simulink model "Robot_Phase1_PASS"  (R2026a)
settings: Solver=ode15s  StopTime=20  FixedStep=0.001  MaxStep=0.01  AbsTol=1e-6
model workspace: external: MATLAB File GDOFrobot_DataFile.m (data not in the file)
values from neighbouring files (symbols this model uses):
  enc_noise_signal = randn(length(t_noise), 3)    [generate_dataset_v2.m]
  N = size(residual, 1)    [extract_features.m]    (also in extract_features_windowed.m)
  t_noise = (0:dt_noise:sim_duration)'    [generate_dataset_v2.m]
  Y = categorical(label_vector)    [SVM_classifier_training.m]
undefined symbols (not defined in the file or in its folder): BEAR_PARAMS, DEG_INDEX, ENC_PARAMS, FAULT_JOINT, FAULT_TYPE, GEAR_PARAMS, IMB_PARAMS, sim_payload_mass, smiData, X, Z
libraries: sm_lib x42, nesl_utility x20, simulink x3
(part 1 of 2)
settings Model: Creator=AMMAR  LastModifiedBy=mkame
settings DebuggingCC: InheritedTsInSrcMsg=none
settings ExplorerConfigSet: InternalSimMechanicsExplorerSettings=|
  | <ExplorerConfiguration>
  | 
  |   <canonicalview>default</canonicalview>
  | 
  |   <TilePanel>
  |     <TileInfo>
  |       <Tiles Columns="1" Count="1" Height="465" Rows="1" Width="822">
  |         <Row Weight="1"/>
  |         <Column Weight="1"/>
  |         <Tile Height="1" Width="1" X="0" Y="0"/>
  |       </Tiles>
  |     </TileInfo>
  |     <SceneInfo>
  |       <SceneViewer>
  |         <IsThisViewStd>
  |           <IsStandardView>off</IsStandardView>
  |           <StandardViewName>Front</StandardViewName>
  |         </IsThisViewStd>
  |         <BGColor>
  |           <R>1</R>
  |           <G>1</G>
  |           <B>1</B>
  |           <A>1</A>
  |         </BGColor>
  |         <Camera>
  |           <DoPerspective>off</DoPerspective>
  |           <Position>
  |             <X>-2.8828618955433565</X>
  |             <Y>-1.823236819125285</Y>
  |             <Z>0.92007110645659929</Z>
  |           </Position>
  |           <Center>
  |             <X>-0.4974271117814994</X>
  |             <Y>-0.23235959407589699</Y>
  |             <Z>0.46408144410745272</Z>
  |           </Center>
  |           <Up>
  |             <X>0.126273929236871</X>
  |             <Y>0.093720705637387533</Y>
  |             <Z>0.98755826366342159</Z>
  |           </Up>
  |           <XLim>0.50845975031305723</XLim>
  |           <YLim>0.50845975031305723</YLim>
  |           <ViewLimDist>0.01</ViewLimDist>
  |         </Camera>
  |       </SceneViewer>
  |     </SceneInfo>
  |   </TilePanel>
  | 
  |   <MechEditorPanel>
  |     <GfxPanelCameraMap/>
  |     <Cameras/>
  |     <VideoCreator>
  |       <IncludeTiles>All</IncludeTiles>
  |       <IncludeTime>on</IncludeTime>
  |       <IncludeWorldFrame>off</IncludeWorldFrame>
  |       <PlaybackSpeedRatio>1</PlaybackSpeedRatio>
  |       <FrameRate>30</FrameRate>
  |       <FrameSize>auto</FrameSize>
  |       <VideoFormat>UncompressedAVI</VideoFormat>
  |     </VideoCreator>
  |   </MechEditorPanel>
  | 
  |   <PlaybackSettings>
  |     <PlaybackSpeedFactor>2</PlaybackSpeedFactor>
  |   </PlaybackSettings>
  | 
  | </ExplorerConfiguration>

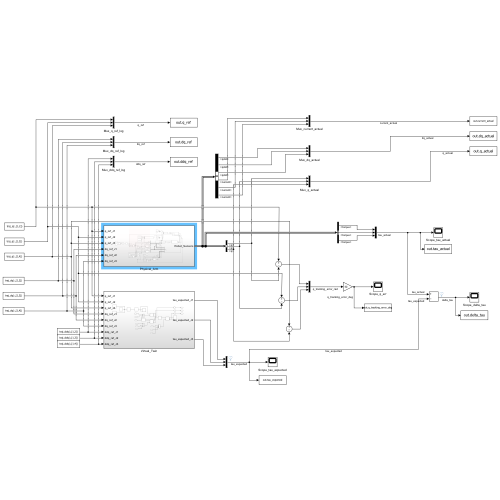
[thumbnail: Simulink's stored preview of the top-level diagram]
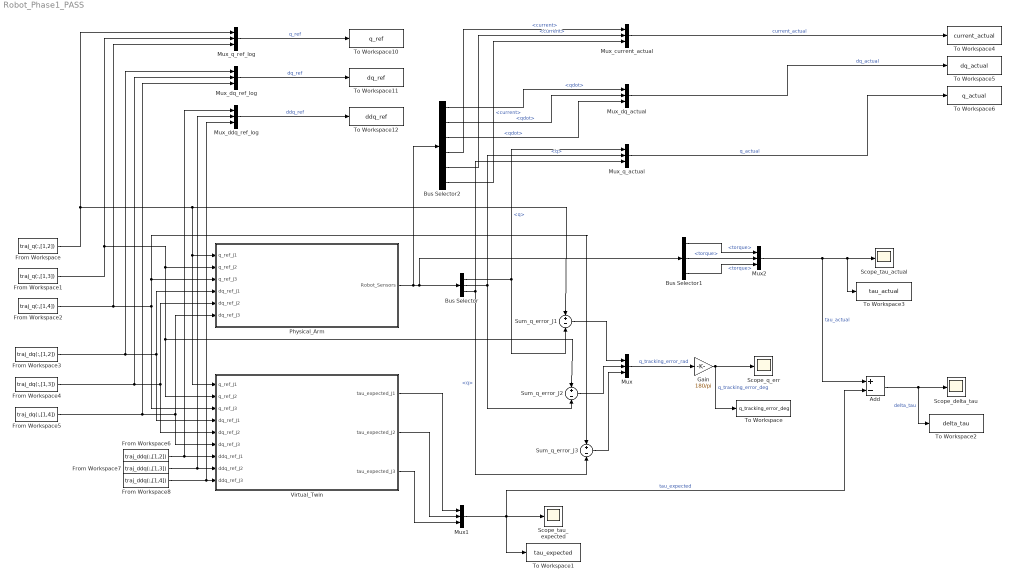
== system Robot_Phase1_PASS ==
  Add : Sum  Inputs=+-
  Bus Selector : BusSelector  OutputSignals=Joint1_Signals.q,Joint2_Signals.q,Joint3_Signals.q
  Bus Selector1 : BusSelector  OutputSignals=Joint1_Signals.torque,Joint2_Signals.torque,Joint3_Signals.torque
  Bus Selector2 : BusSelector  OutputSignals=Joint1_Signals.qdot,Joint2_Signals.qdot,Joint3_Signals.qdot,Joint1_Signals.current,Joint2_Signals.current,Joint3_Signals.current
  From Workspace : FromWorkspace  VariableName=traj_q(:,[1,2])  SampleTime=-1
  From Workspace1 : FromWorkspace  VariableName=traj_q(:,[1,3])  SampleTime=-1
  From Workspace2 : FromWorkspace  VariableName=traj_q(:,[1,4])  SampleTime=-1
  From Workspace3 : FromWorkspace  VariableName=traj_dq(:,[1,2])  SampleTime=-1
  From Workspace4 : FromWorkspace  VariableName=traj_dq(:,[1,3])  SampleTime=-1
  From Workspace5 : FromWorkspace  VariableName=traj_dq(:,[1,4])  SampleTime=-1
  From Workspace6 : FromWorkspace  VariableName=traj_ddq(:,[1,2])  SampleTime=-1
  From Workspace7 : FromWorkspace  VariableName=traj_ddq(:,[1,3])  SampleTime=-1
  From Workspace8 : FromWorkspace  VariableName=traj_ddq(:,[1,4])  SampleTime=-1
  Gain : Gain  Gain=180/pi
  Mux : Mux  Inputs=3
  Mux1 : Mux  Inputs=3
  Mux2 : Mux  Inputs=3
  Mux_current_actual : Mux  Inputs=3
  Mux_ddq_ref_log : Mux  Inputs=3
  Mux_dq_actual : Mux  Inputs=3
  Mux_dq_ref_log : Mux  Inputs=3
  Mux_q_actual : Mux  Inputs=3
  Mux_q_ref_log : Mux  Inputs=3
  Physical_Arm : Subsystem
  Scope_delta_tau : Scope
      settings: ActiveDisplayYMinimum=-2.4660979772206608  ActiveDisplayYMaximum=7.674798064954345  DataLoggingVariableName=ScopeData2
  Scope_q_err : Scope
      settings: ActiveDisplayYMinimum=-97.469420637848955  ActiveDisplayYMaximum=96.880109513754348
  Scope_tau_actual : Scope
      settings: ActiveDisplayYMinimum=-1  ActiveDisplayYMaximum=1  DataLoggingVariableName=ScopeData3
  Scope_tau_expected : Scope
      settings: ActiveDisplayYMinimum=-15.168732068313531  ActiveDisplayYMaximum=6.028938661872969
  "Sum_q_error_J1 " : Sum  Inputs=+-
  Sum_q_error_J2 : Sum  Inputs=+-
  Sum_q_error_J3 : Sum  Inputs=+-
  To Workspace : ToWorkspace  VariableName=q_tracking_error_deg  SaveFormat=Timeseries  SampleTime=-1
  To Workspace1 : ToWorkspace  VariableName=tau_expected  SaveFormat=Timeseries  SampleTime=-1
  To Workspace10 : ToWorkspace  VariableName=q_ref  SaveFormat=Timeseries  SampleTime=-1
  To Workspace11 : ToWorkspace  VariableName=dq_ref  SaveFormat=Timeseries  SampleTime=-1
  To Workspace12 : ToWorkspace  VariableName=ddq_ref  SaveFormat=Timeseries  SampleTime=-1
  To Workspace2 : ToWorkspace  VariableName=delta_tau  SaveFormat=Timeseries  SampleTime=-1
  To Workspace3 : ToWorkspace  VariableName=tau_actual  SaveFormat=Timeseries  SampleTime=-1
  To Workspace4 : ToWorkspace  VariableName=current_actual  SaveFormat=Timeseries  SampleTime=-1
  To Workspace5 : ToWorkspace  VariableName=dq_actual  SaveFormat=Timeseries  SampleTime=-1
  To Workspace6 : ToWorkspace  VariableName=q_actual  SaveFormat=Timeseries  SampleTime=-1
  Virtual_Twin : Subsystem
  wires:
  From Workspace/1 -> Mux_q_ref_log/1, Virtual_Twin/1("q_ref_J1 "), Physical_Arm/1("q_ref_J1  "), "Sum_q_error_J1 "/1
  From Workspace4/1 -> Mux_dq_ref_log/2, Physical_Arm/5(dq_ref_J2), Virtual_Twin/5(dq_ref_J2)
  From Workspace7/1 -> Mux_ddq_ref_log/2, Virtual_Twin/8(ddq_ref_J2)
  From Workspace1/1 -> Mux_q_ref_log/2, Virtual_Twin/2(q_ref_J2), Sum_q_error_J2/1, Physical_Arm/2(q_ref_J2)
  From Workspace5/1 -> Mux_dq_ref_log/3, Physical_Arm/6(dq_ref_J3), Virtual_Twin/6(dq_ref_J3)
  From Workspace3/1 -> Mux_dq_ref_log/1, Physical_Arm/4(dq_ref_J1), Virtual_Twin/4(dq_ref_J1)
  From Workspace2/1 -> Mux_q_ref_log/3, Sum_q_error_J3/1, Physical_Arm/3(q_ref_J3), Virtual_Twin/3(q_ref_J3)
  From Workspace6/1 -> Mux_ddq_ref_log/1, Virtual_Twin/7(ddq_ref_J1)
  From Workspace8/1 -> Mux_ddq_ref_log/3, Virtual_Twin/9(ddq_ref_J3)
  Physical_Arm/1(Robot_Sensors) -> Bus Selector2/1, Bus Selector1/1, Bus Selector/1
  Bus Selector/1 -> Mux_q_actual/1, "Sum_q_error_J1 "/2  "<q>"
  "Sum_q_error_J1 "/1 -> Mux/1
  Sum_q_error_J2/1 -> Mux/2
  Sum_q_error_J3/1 -> Mux/3
  Mux/1 -> Gain/1  "q_tracking_error_rad"
  Gain/1 -> To Workspace/1, Scope_q_err/1  "q_tracking_error_deg"
  Bus Selector/2 -> Mux_q_actual/2, Sum_q_error_J2/2  "<q>"
  Bus Selector/3 -> Mux_q_actual/3, Sum_q_error_J3/2  "<q>"
  Virtual_Twin/1(tau_expected_J1) -> Mux1/1
  Virtual_Twin/2(tau_expected_J2) -> Mux1/2
  Virtual_Twin/3(tau_expected_J3) -> Mux1/3
  Mux1/1 -> To Workspace1/1, Add/2, Scope_tau_expected/1  "tau_expected"
  Bus Selector1/1 -> Mux2/1  "<torque>"
  Bus Selector1/2 -> Mux2/2  "<torque>"
  Bus Selector1/3 -> Mux2/3  "<torque>"
  Mux2/1 -> Add/1, To Workspace3/1, Scope_tau_actual/1  "tau_actual"
  Add/1 -> To Workspace2/1, Scope_delta_tau/1  "delta_tau"
  Bus Selector2/1 -> Mux_dq_actual/1  "<qdot>"
  Bus Selector2/2 -> Mux_dq_actual/2  "<qdot>"
  Bus Selector2/3 -> Mux_dq_actual/3  "<qdot>"
  Bus Selector2/4 -> Mux_current_actual/1  "<current>"
  Bus Selector2/5 -> Mux_current_actual/2  "<current>"
  Bus Selector2/6 -> Mux_current_actual/3  "<current>"
  Mux_current_actual/1 -> To Workspace4/1  "current_actual"
  Mux_dq_actual/1 -> To Workspace5/1  "dq_actual"
  Mux_q_actual/1 -> To Workspace6/1  "q_actual"
  Mux_q_ref_log/1 -> To Workspace10/1  "q_ref"
  Mux_dq_ref_log/1 -> To Workspace11/1  "dq_ref"
  Mux_ddq_ref_log/1 -> To Workspace12/1  "ddq_ref"

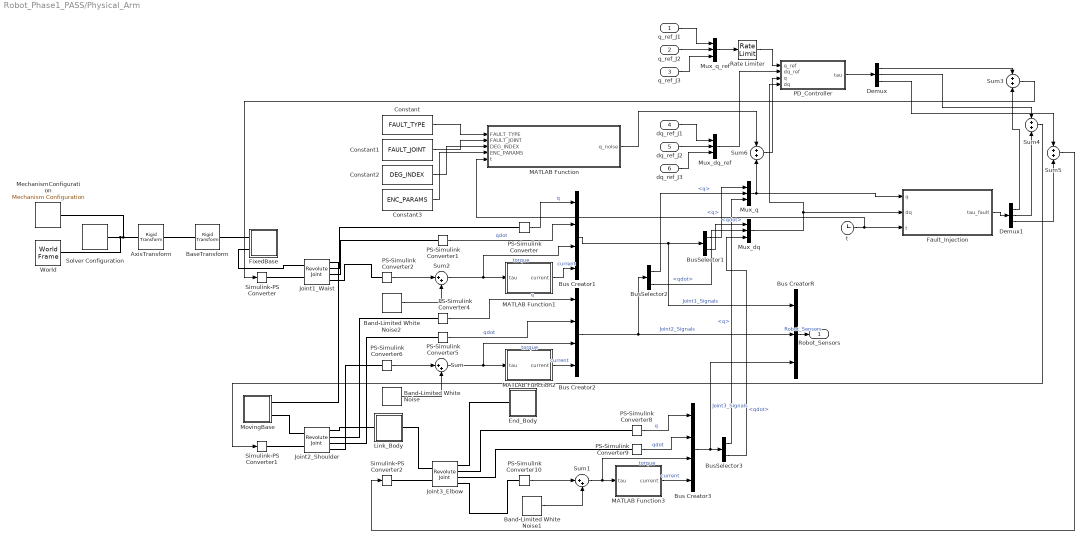
== system Robot_Phase1_PASS/Physical_Arm ==
  "q_ref_J1  " : Inport
  q_ref_J2 : Inport  Port=2
  q_ref_J3 : Inport  Port=3
  dq_ref_J1 : Inport  Port=4
  dq_ref_J2 : Inport  Port=5
  dq_ref_J3 : Inport  Port=6
  AxisTransform : sm_lib/Frames and Transforms/Rigid Transform  RotationMethod=StandardAxis  FollAlignAxisA=+X  BaseAlignAxisA=+Y  FollAlignAxisB=+Y  BaseAlignAxisB=+Z  RotationStandardAxis=+X  RotationAngle=pi/2  RotationAngleUnits=rad  RotationArbitraryAxis=[0 0 1]  RotationSequenceAxes=FollowerAxes  RotationSequence=XYX  RotationSequenceAngles=[0 0 0]  RotationSequenceAnglesUnits=deg  RotationMatrix=[1 0 0;0 1 0;0 0 1]  Quaternion=[1 0 0 0]  TranslationMethod=None  TranslationCartesianOffset=[0 0 0]  TranslationCartesianOffsetUnits=m  TranslationStandardAxis=+Z  TranslationStandardOffset=0  TranslationStandardOffsetUnits=m  TranslationROffset=0  TranslationROffsetUnits=m  TranslationThetaOffset=0  TranslationThetaOffsetUnits=deg  TranslationZOffset=0  TranslationZOffsetUnits=m
  Band-Limited White Noise : simulink/Sources/Band-Limited White Noise  Cov=[1e-7]  Ts=0.001  seed=[23342]
  Band-Limited White Noise1 : simulink/Sources/Band-Limited White Noise  Cov=[1e-7]  Ts=0.001  seed=[23343]
  Band-Limited White Noise2 : simulink/Sources/Band-Limited White Noise  Cov=[1e-7]  Ts=0.001  seed=[23341]
  BaseTransform : sm_lib/Frames and Transforms/Rigid Transform  RotationMethod=ArbitraryAxis  FollAlignAxisA=+X  BaseAlignAxisA=+Y  FollAlignAxisB=+Y  BaseAlignAxisB=+Z  RotationStandardAxis=+X  RotationAngle=smiData.RigidTransform(7).angle  RotationAngleUnits=rad  RotationArbitraryAxis=smiData.RigidTransform(7).axis  RotationSequenceAxes=FollowerAxes  RotationSequence=XYX  RotationSequenceAngles=[0 0 0]  RotationSequenceAnglesUnits=deg  RotationMatrix=[1 0 0;0 1 0;0 0 1]  Quaternion=[1 0 0 0]  TranslationMethod=Cartesian  TranslationCartesianOffset=smiData.RigidTransform(7).translation  TranslationCartesianOffsetUnits=mm  TranslationStandardAxis=+Z  TranslationStandardOffset=0.75  TranslationStandardOffsetUnits=m  TranslationROffset=0  TranslationROffsetUnits=m  TranslationThetaOffset=0  TranslationThetaOffsetUnits=deg  TranslationZOffset=0  TranslationZOffsetUnits=m
  Bus Creator1 : BusCreator  Inputs=4
  Bus Creator2 : BusCreator  Inputs=4
  Bus Creator3 : BusCreator  Inputs=4
  Bus CreatorR : BusCreator  Inputs=3
  BusSelector1 : BusSelector  OutputSignals=q,qdot
  BusSelector2 : BusSelector  OutputSignals=q,qdot
  BusSelector3 : BusSelector  OutputSignals=q,qdot
  Constant : Constant  Value=FAULT_TYPE
  Constant1 : Constant  Value=FAULT_JOINT
  Constant2 : Constant  Value=DEG_INDEX
  Constant3 : Constant  Value=ENC_PARAMS
  Demux : Demux  Outputs=3
  Demux1 : Demux  Outputs=3
  End_Body : Subsystem
  Fault_Injection : Subsystem
  FixedBase : Subsystem
  Joint1_Waist : sm_lib/Joints/Revolute Joint  JointMode=Normal  CompositeWrenchDir=FollowerOnBase  CompositeWrenchFrame=BaseFrame  SenseConstraintForce=off  SenseConstraintTorque=off  SenseTotalForce=off  SenseTotalTorque=off  PositionTargetSpecify=on  PositionTargetPriority=High  PositionTargetValue=0  PositionTargetValueUnits=rad  VelocityTargetSpecify=on  VelocityTargetPriority=High  VelocityTargetValue=0  VelocityTargetValueUnits=deg/s  EquilibriumPosition=0  EquilibriumPositionUnits=deg  SpringStiffness=0  SpringStiffnessUnits=N*m/deg  DampingCoefficient=1  DampingCoefficientUnits=N*m*s/rad  LowerLimitSpecify=on  LowerLimitBound=-180  LowerLimitBoundUnits=deg  LowerLimitStiffness=1e4  LowerLimitStiffnessUnits=N*m/deg  LowerLimitDamping=10  LowerLimitDampingUnits=N*m/(deg/s)  LowerLimitTransitionRegionWidth=0.1  LowerLimitTransitionRegionWidthUnits=deg  UpperLimitSpecify=on  UpperLimitBound=180  UpperLimitBoundUnits=deg  UpperLimitStiffness=1e4  UpperLimitStiffnessUnits=N*m/deg  UpperLimitDamping=10  UpperLimitDampingUnits=N*m/(deg/s)  UpperLimitTransitionRegionWidth=0.1  UpperLimitTransitionRegionWidthUnits=deg  TorqueActuationMode=InputTorque  MotionActuationMode=ComputedMotion  SensePosition=on  SenseVelocity=on  SenseAcceleration=off  SenseTorqueForce=on  SenseLowerLimitTorqueForce=off  SenseUpperLimitTorqueForce=off
  Joint2_Shoulder : sm_lib/Joints/Revolute Joint  JointMode=Normal  CompositeWrenchDir=FollowerOnBase  CompositeWrenchFrame=BaseFrame  SenseConstraintForce=off  SenseConstraintTorque=off  SenseTotalForce=off  SenseTotalTorque=off  PositionTargetSpecify=on  PositionTargetPriority=High  PositionTargetValue=-pi/4  PositionTargetValueUnits=rad  VelocityTargetSpecify=on  VelocityTargetPriority=High  VelocityTargetValue=0  VelocityTargetValueUnits=deg/s  EquilibriumPosition=0  EquilibriumPositionUnits=deg  SpringStiffness=0  SpringStiffnessUnits=N*m/deg  DampingCoefficient=1.5  DampingCoefficientUnits=N*m*s/rad  LowerLimitSpecify=on  LowerLimitBound=-195  LowerLimitBoundUnits=deg  LowerLimitStiffness=1e4  LowerLimitStiffnessUnits=N*m/deg  LowerLimitDamping=10  LowerLimitDampingUnits=N*m/(deg/s)  LowerLimitTransitionRegionWidth=0.1  LowerLimitTransitionRegionWidthUnits=deg  UpperLimitSpecify=on  UpperLimitBound=-15  UpperLimitBoundUnits=deg  UpperLimitStiffness=1e4  UpperLimitStiffnessUnits=N*m/deg  UpperLimitDamping=10  UpperLimitDampingUnits=N*m/(deg/s)  UpperLimitTransitionRegionWidth=0.1  UpperLimitTransitionRegionWidthUnits=deg  TorqueActuationMode=InputTorque  MotionActuationMode=ComputedMotion  SensePosition=on  SenseVelocity=on  SenseAcceleration=off  SenseTorqueForce=on  SenseLowerLimitTorqueForce=off  SenseUpperLimitTorqueForce=off
  Joint3_Elbow : sm_lib/Joints/Revolute Joint  JointMode=Normal  CompositeWrenchDir=FollowerOnBase  CompositeWrenchFrame=BaseFrame  SenseConstraintForce=off  SenseConstraintTorque=off  SenseTotalForce=off  SenseTotalTorque=off  PositionTargetSpecify=on  PositionTargetPriority=High  PositionTargetValue=-pi/4  PositionTargetValueUnits=rad  VelocityTargetSpecify=on  VelocityTargetPriority=High  VelocityTargetValue=0  VelocityTargetValueUnits=deg/s  EquilibriumPosition=0  EquilibriumPositionUnits=deg  SpringStiffness=0  SpringStiffnessUnits=N*m/deg  DampingCoefficient=0.5  DampingCoefficientUnits=N*m*s/rad  LowerLimitSpecify=on  LowerLimitBound=-165  LowerLimitBoundUnits=deg  LowerLimitStiffness=1e4  LowerLimitStiffnessUnits=N*m/deg  LowerLimitDamping=10  LowerLimitDampingUnits=N*m/(deg/s)  LowerLimitTransitionRegionWidth=0.1  LowerLimitTransitionRegionWidthUnits=deg  UpperLimitSpecify=on  UpperLimitBound=60  UpperLimitBoundUnits=deg  UpperLimitStiffness=1e4  UpperLimitStiffnessUnits=N*m/deg  UpperLimitDamping=10  UpperLimitDampingUnits=N*m/(deg/s)  UpperLimitTransitionRegionWidth=0.1  UpperLimitTransitionRegionWidthUnits=deg  TorqueActuationMode=InputTorque  MotionActuationMode=ComputedMotion  SensePosition=on  SenseVelocity=on  SenseAcceleration=off  SenseTorqueForce=on  SenseLowerLimitTorqueForce=off  SenseUpperLimitTorqueForce=off
  Link_Body : Subsystem
  MATLAB Function : MATLAB Function  TreatAsAtomicUnit=on
  MATLAB Function1 : MATLAB Function  TreatAsAtomicUnit=on
  MATLAB Function2 : MATLAB Function  TreatAsAtomicUnit=on
  MATLAB Function3 : MATLAB Function  TreatAsAtomicUnit=on
  MechanismConfiguration : sm_lib/Utilities/Mechanism Configuration  UniformGravity=Constant  GravityVector=[0 0 -9.80665]  GravityVectorUnits=m/s^2  LinearizationDelta=0.001  JointModeTransitionNonlinearIterations=2
  MovingBase : Subsystem
  "Mux_dq   " : Mux  Inputs=3
  "Mux_dq_ref " : Mux  Inputs=3
  "Mux_q    " : Mux  Inputs=3
  "Mux_q_ref  " : Mux  Inputs=3
  PD_Controller : Subsystem
  PS-Simulink Converter : nesl_utility/PS-Simulink Converter  PhysicalDomain=network_engine_domain  SubClassName=ps_output  LeftPortType=input  RightPortType=output  PseudoPeriodic=off  Frequencies=[]  VectorFormat=inherit  Unit=rad  AffineConversion=off
  PS-Simulink Converter{1..2,5..6,9..10} (6 alike) : nesl_utility/PS-Simulink Converter  PhysicalDomain=network_engine_domain  SubClassName=ps_output  LeftPortType=input  RightPortType=output  PseudoPeriodic=off  Frequencies=[]  VectorFormat=inherit  Unit=inherit  AffineConversion=off
  PS-Simulink Converter4 : nesl_utility/PS-Simulink Converter  PhysicalDomain=network_engine_domain  SubClassName=ps_output  LeftPortType=input  RightPortType=output  PseudoPeriodic=off  Frequencies=[]  VectorFormat=inherit  Unit=rad  AffineConversion=off
  PS-Simulink Converter8 : nesl_utility/PS-Simulink Converter  PhysicalDomain=network_engine_domain  SubClassName=ps_output  LeftPortType=input  RightPortType=output  PseudoPeriodic=off  Frequencies=[]  VectorFormat=inherit  Unit=rad  AffineConversion=off
  Rate Limiter : RateLimiter  RisingSlewLimit=10  FallingSlewLimit=-10  SampleTimeMode=inherited
  Simulink-PS Converter : nesl_utility/Simulink-PS Converter  PhysicalDomain=network_engine_domain  SubClassName=ps_input  LeftPortType=input  RightPortType=output  PseudoPeriodic=off  Frequencies=[]  NoiseDistribution=none  NoiseParameters=[]  Unit=N*m  AffineConversion=off  FilteringAndDerivatives=provide  SimscapeFilterOrder=1  InputFilterTimeConstant=0.001  UdotUserProvided=0
  Simulink-PS Converter1 : nesl_utility/Simulink-PS Converter  PhysicalDomain=network_engine_domain  SubClassName=ps_input  LeftPortType=input  RightPortType=output  PseudoPeriodic=off  Frequencies=[]  NoiseDistribution=none  NoiseParameters=[]  Unit=N*m  AffineConversion=off  FilteringAndDerivatives=provide  SimscapeFilterOrder=1  InputFilterTimeConstant=0.001  UdotUserProvided=0
  Simulink-PS Converter2 : nesl_utility/Simulink-PS Converter  PhysicalDomain=network_engine_domain  SubClassName=ps_input  LeftPortType=input  RightPortType=output  PseudoPeriodic=off  Frequencies=[]  NoiseDistribution=none  NoiseParameters=[]  Unit=N*m  AffineConversion=off  FilteringAndDerivatives=provide  SimscapeFilterOrder=1  InputFilterTimeConstant=0.001  UdotUserProvided=0
  Solver Configuration : nesl_utility/Solver Configuration  PhysicalDomain=network_engine_domain  SubClassName=solver  LeftPortType=input  RightPortType=generic  Tones=[]  Harmonics=[]  SimulateNoise=off  Profile=off  UseLocalSampling=off  EnableSwitchedLinearOptims=on  FrequencyDomain=off  UseCCode=off  RelTol=0.001  AbsTol=0.001  MinStep=1e-09  ToWorkspace=off  RevertToSquareIcSolve=off  NumHomotopyIterations=100  PhasorMode=off  PhasorModeNumHarmonics=1  ConsistencySolver=NEWTON_XTOL_AFTER_FTOL  CanonicalOrdering=CANONICAL  OptimizeIntermediates=OPTIMIZED  IndexReductionMethod=DerivativeReplacement  DoDC=off  ResidualTolerance=1e-09  ConsistencyTolSource=GLOBAL  ConsistencyAbsTol=0.001  ConsistencyRelTol=0.001  ConsistencyTolFactor=0.001  UseLocalSolver=off  LocalSolverChoice=NE_BACKWARD_EULER_ADVANCER  ResolveIndetEquations=on  FunctionEvalNumThread=1  LocalSolverSampleTime=0.001  DoFixedCost=off  MaxNonlinIter=3  MaxModeIter=2  ComputeImpulses=off  ImpulseIterations=2  LinearAlgebra=auto  LinearAlgebraNumThread=0  EquationFormulation=NE_TIME_EF  DelaysMemoryBudget=1024  AutomaticFiltering=on  FilteringTimeConstant=0.001  PartitionStorageMethod=AS_NEEDED  PartitionMemoryBudget=1024  PartitionMethod=ROBUST  MultibodyUseLocalSolver=off  MultibodyLocalSolverChoice=ODE1  MultibodyLocalSolverSampleTime=0.001
  Sum : Sum  Inputs=|++
  Sum1 : Sum  Inputs=|++
  Sum2 : Sum  Inputs=|++
  Sum{3..6} (4 alike) : Sum
  World : sm_lib/Frames and Transforms/World Frame
  t : Clock
  Robot_Sensors : Outport
  wires:
  PD_Controller/1(tau) -> Demux/1
  Sum1/1 -> Bus Creator3/3, MATLAB Function3/1(tau)  "torque"
  MATLAB Function2/1(current) -> Bus Creator2/4  "current"
  BusSelector2/2 -> "Mux_dq   "/2  "<qdot>"
  PS-Simulink Converter9/1 -> Bus Creator3/2  "qdot"
  PS-Simulink Converter6/1 -> Sum/1
  Bus Creator2/1 -> BusSelector2/1, Bus CreatorR/2  "Joint2_Signals"
  Rate Limiter/1 -> PD_Controller/1(q_ref)
  Sum2/1 -> Bus Creator1/3, MATLAB Function1/1(tau)  "torque"
  Bus Creator1/1 -> BusSelector1/1, Bus CreatorR/1  "Joint1_Signals"
  BusSelector3/1 -> "Mux_q    "/3  "<q>"
  PS-Simulink Converter2/1 -> Sum2/1
  MATLAB Function1/1(current) -> Bus Creator1/4  "current"
  BusSelector1/2 -> "Mux_dq   "/1  "<qdot>"
  BusSelector1/1 -> "Mux_q    "/1  "<q>"
  Sum/1 -> Bus Creator2/3, MATLAB Function2/1(tau)  "torque"
  PS-Simulink Converter1/1 -> Bus Creator1/2  "qdot"
  PS-Simulink Converter8/1 -> Bus Creator3/1  "q"
  BusSelector2/1 -> "Mux_q    "/2  "<q>"
  "Mux_dq   "/1 -> PD_Controller/4(dq), Fault_Injection/2(dq)
  Bus CreatorR/1 -> Robot_Sensors/1  "Robot_Sensors"
  PS-Simulink Converter4/1 -> Bus Creator2/1  "q"
  PS-Simulink Converter5/1 -> Bus Creator2/2  "qdot"
  Bus Creator3/1 -> Bus CreatorR/3, BusSelector3/1  "Joint3_Signals"
  Band-Limited White Noise/1 -> Sum/2
  BusSelector3/2 -> "Mux_dq   "/3  "<qdot>"
  PS-Simulink Converter10/1 -> Sum1/1
  MATLAB Function3/1(current) -> Bus Creator3/4  "current"
  "Mux_dq_ref "/1 -> PD_Controller/2(dq_ref)
  Band-Limited White Noise1/1 -> Sum1/2
  "Mux_q    "/1 -> Fault_Injection/1(q), Sum6/2
  Band-Limited White Noise2/1 -> Sum2/2
  "Mux_q_ref  "/1 -> Rate Limiter/1
  PS-Simulink Converter/1 -> Bus Creator1/1  "q"
  "q_ref_J1  "/1 -> "Mux_q_ref  "/1
  q_ref_J2/1 -> "Mux_q_ref  "/2
  q_ref_J3/1 -> "Mux_q_ref  "/3
  dq_ref_J1/1 -> "Mux_dq_ref "/1
  dq_ref_J2/1 -> "Mux_dq_ref "/2
  dq_ref_J3/1 -> "Mux_dq_ref "/3
  t/1 -> MATLAB Function/5(t), Fault_Injection/3(t)
  Fault_Injection/1(tau_fault) -> Demux1/1
  Demux/1 -> Sum3/1
  Demux1/1 -> Sum3/2
  Demux/2 -> Sum4/1
  Demux1/2 -> Sum4/2
  Demux1/3 -> Sum5/2
  Demux/3 -> Sum5/1
  Sum3/1 -> Simulink-PS Converter/1
  Sum4/1 -> Simulink-PS Converter1/1
  Sum5/1 -> Simulink-PS Converter2/1
  Sum6/1 -> PD_Controller/3(q)
  MATLAB Function/1(q_noise) -> Sum6/1
  Constant/1 -> MATLAB Function/1(FAULT_TYPE)
  Constant1/1 -> MATLAB Function/2(FAULT_JOINT)
  Constant2/1 -> MATLAB Function/3(DEG_INDEX)
  Constant3/1 -> MATLAB Function/4(ENC_PARAMS)
  connections:
  Joint1_Waist/RConn3 -- PS-Simulink Converter1/LConn1
  Joint1_Waist/RConn4 -- PS-Simulink Converter2/LConn1
  Joint3_Elbow/RConn4 -- PS-Simulink Converter10/LConn1
  MovingBase/RConn2 -- Joint2_Shoulder/LConn1
  Solver Configuration/RConn1 -- AxisTransform/LConn1 -- MechanismConfiguration/RConn1 -- World/RConn1
  Joint1_Waist/LConn2 -- Simulink-PS Converter/RConn1
  Joint3_Elbow/LConn2 -- Simulink-PS Converter2/RConn1
  Joint2_Shoulder/RConn4 -- PS-Simulink Converter6/LConn1
  BaseTransform/RConn1 -- FixedBase/LConn1
  AxisTransform/RConn1 -- BaseTransform/LConn1
  Joint2_Shoulder/RConn2 -- PS-Simulink Converter4/LConn1
  Joint1_Waist/RConn2 -- PS-Simulink Converter/LConn1
  MovingBase/RConn1 -- Joint1_Waist/RConn1
  FixedBase/LConn2 -- Joint1_Waist/LConn1
  Joint2_Shoulder/RConn1 -- Link_Body/LConn1
  Link_Body/RConn1 -- Joint3_Elbow/LConn1
  Joint3_Elbow/RConn1 -- End_Body/LConn1
  Simulink-PS Converter1/RConn1 -- Joint2_Shoulder/LConn2
  Joint3_Elbow/RConn3 -- PS-Simulink Converter9/LConn1
  Joint3_Elbow/RConn2 -- PS-Simulink Converter8/LConn1
  Joint2_Shoulder/RConn3 -- PS-Simulink Converter5/LConn1

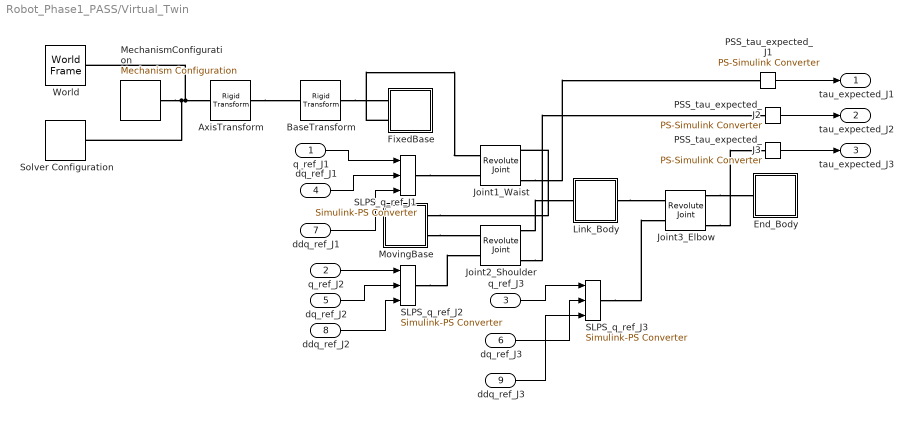
== system Robot_Phase1_PASS/Virtual_Twin ==
  "q_ref_J1 " : Inport
  q_ref_J2 : Inport  Port=2
  q_ref_J3 : Inport  Port=3
  dq_ref_J1 : Inport  Port=4
  dq_ref_J2 : Inport  Port=5
  dq_ref_J3 : Inport  Port=6
  ddq_ref_J1 : Inport  Port=7
  ddq_ref_J2 : Inport  Port=8
  ddq_ref_J3 : Inport  Port=9
  AxisTransform : sm_lib/Frames and Transforms/Rigid Transform  RotationMethod=StandardAxis  FollAlignAxisA=+X  BaseAlignAxisA=+Y  FollAlignAxisB=+Y  BaseAlignAxisB=+Z  RotationStandardAxis=+X  RotationAngle=pi/2  RotationAngleUnits=rad  RotationArbitraryAxis=[0 0 1]  RotationSequenceAxes=FollowerAxes  RotationSequence=XYX  RotationSequenceAngles=[0 0 0]  RotationSequenceAnglesUnits=deg  RotationMatrix=[1 0 0;0 1 0;0 0 1]  Quaternion=[1 0 0 0]  TranslationMethod=None  TranslationCartesianOffset=[0 0 0]  TranslationCartesianOffsetUnits=m  TranslationStandardAxis=+Z  TranslationStandardOffset=0  TranslationStandardOffsetUnits=m  TranslationROffset=0  TranslationROffsetUnits=m  TranslationThetaOffset=0  TranslationThetaOffsetUnits=deg  TranslationZOffset=0  TranslationZOffsetUnits=m
  BaseTransform : sm_lib/Frames and Transforms/Rigid Transform  RotationMethod=ArbitraryAxis  FollAlignAxisA=+X  BaseAlignAxisA=+Y  FollAlignAxisB=+Y  BaseAlignAxisB=+Z  RotationStandardAxis=+X  RotationAngle=smiData.RigidTransform(7).angle  RotationAngleUnits=rad  RotationArbitraryAxis=smiData.RigidTransform(7).axis  RotationSequenceAxes=FollowerAxes  RotationSequence=XYX  RotationSequenceAngles=[0 0 0]  RotationSequenceAnglesUnits=deg  RotationMatrix=[1 0 0;0 1 0;0 0 1]  Quaternion=[1 0 0 0]  TranslationMethod=Cartesian  TranslationCartesianOffset=smiData.RigidTransform(7).translation  TranslationCartesianOffsetUnits=mm  TranslationStandardAxis=+Z  TranslationStandardOffset=0.75  TranslationStandardOffsetUnits=m  TranslationROffset=0  TranslationROffsetUnits=m  TranslationThetaOffset=0  TranslationThetaOffsetUnits=deg  TranslationZOffset=0  TranslationZOffsetUnits=m
  End_Body : Subsystem
  FixedBase : Subsystem
  Joint1_Waist : sm_lib/Joints/Revolute Joint  JointMode=Normal  CompositeWrenchDir=FollowerOnBase  CompositeWrenchFrame=BaseFrame  SenseConstraintForce=off  SenseConstraintTorque=off  SenseTotalForce=off  SenseTotalTorque=off  PositionTargetSpecify=on  PositionTargetPriority=High  PositionTargetValue=0  PositionTargetValueUnits=rad  VelocityTargetSpecify=on  VelocityTargetPriority=High  VelocityTargetValue=0  VelocityTargetValueUnits=deg/s  EquilibriumPosition=0  EquilibriumPositionUnits=deg  SpringStiffness=0  SpringStiffnessUnits=N*m/deg  DampingCoefficient=0  DampingCoefficientUnits=N*m*s/rad  LowerLimitSpecify=off  LowerLimitBound=-180  LowerLimitBoundUnits=deg  LowerLimitStiffness=1e4  LowerLimitStiffnessUnits=N*m/deg  LowerLimitDamping=10  LowerLimitDampingUnits=N*m/(deg/s)  LowerLimitTransitionRegionWidth=0.1  LowerLimitTransitionRegionWidthUnits=deg  UpperLimitSpecify=off  UpperLimitBound=180  UpperLimitBoundUnits=deg  UpperLimitStiffness=1e4  UpperLimitStiffnessUnits=N*m/deg  UpperLimitDamping=10  UpperLimitDampingUnits=N*m/(deg/s)  UpperLimitTransitionRegionWidth=0.1  UpperLimitTransitionRegionWidthUnits=deg  TorqueActuationMode=ComputedTorque  MotionActuationMode=InputMotion  SensePosition=on  SenseVelocity=on  SenseAcceleration=off  SenseTorqueForce=on  SenseLowerLimitTorqueForce=off  SenseUpperLimitTorqueForce=off
  Joint2_Shoulder : sm_lib/Joints/Revolute Joint  JointMode=Normal  CompositeWrenchDir=FollowerOnBase  CompositeWrenchFrame=BaseFrame  SenseConstraintForce=off  SenseConstraintTorque=off  SenseTotalForce=off  SenseTotalTorque=off  PositionTargetSpecify=on  PositionTargetPriority=High  PositionTargetValue=-pi/4  PositionTargetValueUnits=rad  VelocityTargetSpecify=on  VelocityTargetPriority=High  VelocityTargetValue=0  VelocityTargetValueUnits=deg/s  EquilibriumPosition=0  EquilibriumPositionUnits=deg  SpringStiffness=0  SpringStiffnessUnits=N*m/deg  DampingCoefficient=0  DampingCoefficientUnits=N*m*s/rad  LowerLimitSpecify=off  LowerLimitBound=-195  LowerLimitBoundUnits=deg  LowerLimitStiffness=1e4  LowerLimitStiffnessUnits=N*m/deg  LowerLimitDamping=10  LowerLimitDampingUnits=N*m/(deg/s)  LowerLimitTransitionRegionWidth=0.1  LowerLimitTransitionRegionWidthUnits=deg  UpperLimitSpecify=off  UpperLimitBound=-15  UpperLimitBoundUnits=deg  UpperLimitStiffness=1e4  UpperLimitStiffnessUnits=N*m/deg  UpperLimitDamping=10  UpperLimitDampingUnits=N*m/(deg/s)  UpperLimitTransitionRegionWidth=0.1  UpperLimitTransitionRegionWidthUnits=deg  TorqueActuationMode=ComputedTorque  MotionActuationMode=InputMotion  SensePosition=on  SenseVelocity=on  SenseAcceleration=off  SenseTorqueForce=on  SenseLowerLimitTorqueForce=off  SenseUpperLimitTorqueForce=off
  Joint3_Elbow : sm_lib/Joints/Revolute Joint  JointMode=Normal  CompositeWrenchDir=FollowerOnBase  CompositeWrenchFrame=BaseFrame  SenseConstraintForce=off  SenseConstraintTorque=off  SenseTotalForce=off  SenseTotalTorque=off  PositionTargetSpecify=on  PositionTargetPriority=High  PositionTargetValue=-pi/4  PositionTargetValueUnits=rad  VelocityTargetSpecify=on  VelocityTargetPriority=High  VelocityTargetValue=0  VelocityTargetValueUnits=deg/s  EquilibriumPosition=0  EquilibriumPositionUnits=deg  SpringStiffness=0  SpringStiffnessUnits=N*m/deg  DampingCoefficient=0  DampingCoefficientUnits=N*m*s/rad  LowerLimitSpecify=off  LowerLimitBound=-165  LowerLimitBoundUnits=deg  LowerLimitStiffness=1e4  LowerLimitStiffnessUnits=N*m/deg  LowerLimitDamping=10  LowerLimitDampingUnits=N*m/(deg/s)  LowerLimitTransitionRegionWidth=0.1  LowerLimitTransitionRegionWidthUnits=deg  UpperLimitSpecify=off  UpperLimitBound=60  UpperLimitBoundUnits=deg  UpperLimitStiffness=1e4  UpperLimitStiffnessUnits=N*m/deg  UpperLimitDamping=10  UpperLimitDampingUnits=N*m/(deg/s)  UpperLimitTransitionRegionWidth=0.1  UpperLimitTransitionRegionWidthUnits=deg  TorqueActuationMode=ComputedTorque  MotionActuationMode=InputMotion  SensePosition=on  SenseVelocity=on  SenseAcceleration=off  SenseTorqueForce=on  SenseLowerLimitTorqueForce=off  SenseUpperLimitTorqueForce=off
  Link_Body : Subsystem
  MechanismConfiguration : sm_lib/Utilities/Mechanism Configuration  UniformGravity=Constant  GravityVector=[0 0 -9.80665]  GravityVectorUnits=m/s^2  LinearizationDelta=0.001  JointModeTransitionNonlinearIterations=2
  MovingBase : Subsystem
  PSS_tau_expected_J1 : nesl_utility/PS-Simulink Converter  PhysicalDomain=network_engine_domain  SubClassName=ps_output  LeftPortType=input  RightPortType=output  PseudoPeriodic=off  Frequencies=[]  VectorFormat=inherit  Unit=N*m  AffineConversion=off
  PSS_tau_expected_J2 : nesl_utility/PS-Simulink Converter  PhysicalDomain=network_engine_domain  SubClassName=ps_output  LeftPortType=input  RightPortType=output  PseudoPeriodic=off  Frequencies=[]  VectorFormat=inherit  Unit=N*m  AffineConversion=off
  PSS_tau_expected_J3 : nesl_utility/PS-Simulink Converter  PhysicalDomain=network_engine_domain  SubClassName=ps_output  LeftPortType=input  RightPortType=output  PseudoPeriodic=off  Frequencies=[]  VectorFormat=inherit  Unit=N*m  AffineConversion=off
  "SLPS_q_ref_J1 " : nesl_utility/Simulink-PS Converter  PhysicalDomain=network_engine_domain  SubClassName=ps_input  LeftPortType=input  RightPortType=output  PseudoPeriodic=off  Frequencies=[]  NoiseDistribution=none  NoiseParameters=[]  Unit=rad  AffineConversion=off  FilteringAndDerivatives=provide  SimscapeFilterOrder=2  InputFilterTimeConstant=0.001  UdotUserProvided=2
  SLPS_q_ref_J2 : nesl_utility/Simulink-PS Converter  PhysicalDomain=network_engine_domain  SubClassName=ps_input  LeftPortType=input  RightPortType=output  PseudoPeriodic=off  Frequencies=[]  NoiseDistribution=none  NoiseParameters=[]  Unit=rad  AffineConversion=off  FilteringAndDerivatives=provide  SimscapeFilterOrder=1  InputFilterTimeConstant=0.001  UdotUserProvided=2
  SLPS_q_ref_J3 : nesl_utility/Simulink-PS Converter  PhysicalDomain=network_engine_domain  SubClassName=ps_input  LeftPortType=input  RightPortType=output  PseudoPeriodic=off  Frequencies=[]  NoiseDistribution=none  NoiseParameters=[]  Unit=rad  AffineConversion=off  FilteringAndDerivatives=provide  SimscapeFilterOrder=1  InputFilterTimeConstant=0.001  UdotUserProvided=2
  Solver Configuration : nesl_utility/Solver Configuration  PhysicalDomain=network_engine_domain  SubClassName=solver  LeftPortType=input  RightPortType=generic  Tones=[]  Harmonics=[]  SimulateNoise=off  Profile=off  UseLocalSampling=off  EnableSwitchedLinearOptims=on  FrequencyDomain=off  UseCCode=off  RelTol=0.001  AbsTol=0.001  MinStep=1e-09  ToWorkspace=off  RevertToSquareIcSolve=off  NumHomotopyIterations=100  PhasorMode=off  PhasorModeNumHarmonics=1  ConsistencySolver=NEWTON_XTOL_AFTER_FTOL  CanonicalOrdering=CANONICAL  OptimizeIntermediates=OPTIMIZED  IndexReductionMethod=DerivativeReplacement  DoDC=off  ResidualTolerance=1e-09  ConsistencyTolSource=GLOBAL  ConsistencyAbsTol=0.001  ConsistencyRelTol=0.001  ConsistencyTolFactor=0.001  UseLocalSolver=off  LocalSolverChoice=NE_BACKWARD_EULER_ADVANCER  ResolveIndetEquations=on  FunctionEvalNumThread=1  LocalSolverSampleTime=0.001  DoFixedCost=off  MaxNonlinIter=3  MaxModeIter=2  ComputeImpulses=off  ImpulseIterations=2  LinearAlgebra=auto  LinearAlgebraNumThread=0  EquationFormulation=NE_TIME_EF  DelaysMemoryBudget=1024  AutomaticFiltering=on  FilteringTimeConstant=0.001  PartitionStorageMethod=AS_NEEDED  PartitionMemoryBudget=1024  PartitionMethod=ROBUST  MultibodyUseLocalSolver=off  MultibodyLocalSolverChoice=ODE1  MultibodyLocalSolverSampleTime=0.001
  World : sm_lib/Frames and Transforms/World Frame
  tau_expected_J1 : Outport
  tau_expected_J2 : Outport  Port=2
  tau_expected_J3 : Outport  Port=3
  wires:
  q_ref_J2/1 -> SLPS_q_ref_J2/1
  "q_ref_J1 "/1 -> "SLPS_q_ref_J1 "/1
  q_ref_J3/1 -> SLPS_q_ref_J3/1
  dq_ref_J1/1 -> "SLPS_q_ref_J1 "/2
  ddq_ref_J1/1 -> "SLPS_q_ref_J1 "/3
  dq_ref_J2/1 -> SLPS_q_ref_J2/2
  ddq_ref_J2/1 -> SLPS_q_ref_J2/3
  dq_ref_J3/1 -> SLPS_q_ref_J3/2
  ddq_ref_J3/1 -> SLPS_q_ref_J3/3
  PSS_tau_expected_J1/1 -> tau_expected_J1/1
  PSS_tau_expected_J2/1 -> tau_expected_J2/1
  PSS_tau_expected_J3/1 -> tau_expected_J3/1
  connections:
  MechanismConfiguration/RConn1 -- AxisTransform/LConn1 -- World/RConn1 -- Solver Configuration/RConn1
  Joint2_Shoulder/RConn4 -- PSS_tau_expected_J2/LConn1
  "SLPS_q_ref_J1 "/RConn1 -- Joint1_Waist/LConn2
  AxisTransform/RConn1 -- BaseTransform/LConn1
  FixedBase/LConn2 -- Joint1_Waist/LConn1
  BaseTransform/RConn1 -- FixedBase/LConn1
  MovingBase/RConn1 -- Joint1_Waist/RConn1
  MovingBase/RConn2 -- Joint2_Shoulder/LConn1
  SLPS_q_ref_J2/RConn1 -- Joint2_Shoulder/LConn2
  Joint2_Shoulder/RConn1 -- Link_Body/LConn1
  Link_Body/RConn1 -- Joint3_Elbow/LConn1
  SLPS_q_ref_J3/RConn1 -- Joint3_Elbow/LConn2
  Joint3_Elbow/RConn1 -- End_Body/LConn1
  Joint3_Elbow/RConn4 -- PSS_tau_expected_J3/LConn1
  Joint1_Waist/RConn4 -- PSS_tau_expected_J1/LConn1

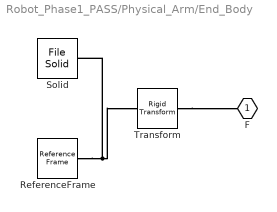
== system Robot_Phase1_PASS/Physical_Arm/End_Body ==
  ReferenceFrame : sm_lib/Frames and Transforms/Reference Frame
  Solid : sm_lib/Body Elements/File Solid  ExtGeomFileName=Link2_Default_sldprt.STEP  UnitType=FromFile  ExtGeomFileUnits=m  StepReaderType=HEX  ExportConvexHullGeometry=off  InertiaType=Custom  BasedOnType=DensityFromFile  Density=1000  DensityUnits=kg/m^3  Mass=sim_payload_mass  MassUnits=kg  CenterOfMass=[0, 0, 0]  CenterOfMassUnits=mm  MomentsOfInertia=[500, 500, 500]  MomentsOfInertiaUnits=kg*mm^2  ProductsOfInertia=[0, 0, 0]  ProductsOfInertiaUnits=kg*mm^2  GraphicType=FromGeometry  MarkerShape=Sphere  MarkerSize=10  GraphicVisPropType=SimpleVisualProperties  GraphicDiffuseColor=smiData.Solid(2).color  GraphicOpacity=smiData.Solid(2).opacity  GraphicSpecularColor=[0.5 0.5 0.5 1.0]  GraphicAmbientColor=[0.15 0.15 0.15 1.0]  GraphicEmissiveColor=[0.0 0.0 0.0 1.0]  GraphicShininess=75  DoExposeReferenceFrame=on  SerializedFrames=<Frames/>
  Transform : sm_lib/Frames and Transforms/Rigid Transform  RotationMethod=ArbitraryAxis  FollAlignAxisA=+X  BaseAlignAxisA=+Y  FollAlignAxisB=+Y  BaseAlignAxisB=+Z  RotationStandardAxis=+X  RotationAngle=smiData.RigidTransform(2).angle  RotationAngleUnits=rad  RotationArbitraryAxis=smiData.RigidTransform(2).axis  RotationSequenceAxes=FollowerAxes  RotationSequence=XYX  RotationSequenceAngles=[0 0 0]  RotationSequenceAnglesUnits=deg  RotationMatrix=[1 0 0;0 1 0;0 0 1]  Quaternion=[1 0 0 0]  TranslationMethod=Cartesian  TranslationCartesianOffset=smiData.RigidTransform(2).translation  TranslationCartesianOffsetUnits=mm  TranslationStandardAxis=+Z  TranslationStandardOffset=0  TranslationStandardOffsetUnits=m  TranslationROffset=0  TranslationROffsetUnits=m  TranslationThetaOffset=0  TranslationThetaOffsetUnits=deg  TranslationZOffset=0  TranslationZOffsetUnits=m
  F : PMIOPort  Side=Left
  connections:
  Solid/RConn1 -- ReferenceFrame/RConn1 -- Transform/LConn1
  Transform/RConn1 -- F/RConn1

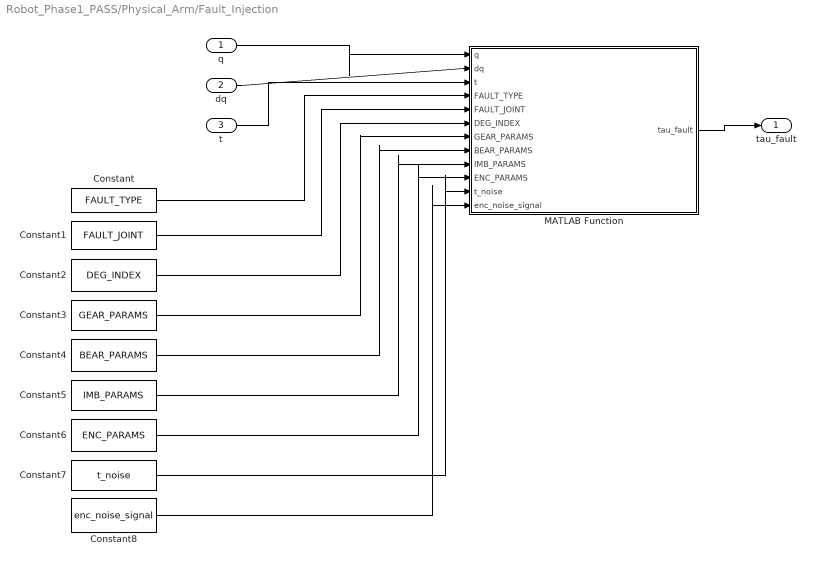
== system Robot_Phase1_PASS/Physical_Arm/Fault_Injection ==
  q : Inport
  dq : Inport  Port=2
  t : Inport  Port=3
  Constant : Constant  Value=FAULT_TYPE
  Constant1 : Constant  Value=FAULT_JOINT
  Constant2 : Constant  Value=DEG_INDEX
  Constant3 : Constant  Value=GEAR_PARAMS
  Constant4 : Constant  Value=BEAR_PARAMS
  Constant5 : Constant  Value=IMB_PARAMS
  Constant6 : Constant  Value=ENC_PARAMS
  Constant7 : Constant  Value=t_noise
  Constant8 : Constant  Value=enc_noise_signal
  MATLAB Function : MATLAB Function  TreatAsAtomicUnit=on
  tau_fault : Outport
  wires:
  q/1 -> MATLAB Function/1(q)
  dq/1 -> MATLAB Function/2(dq)
  t/1 -> MATLAB Function/3(t)
  MATLAB Function/1(tau_fault) -> tau_fault/1
  Constant/1 -> MATLAB Function/4(FAULT_TYPE)
  Constant1/1 -> MATLAB Function/5(FAULT_JOINT)
  Constant2/1 -> MATLAB Function/6(DEG_INDEX)
  Constant3/1 -> MATLAB Function/7(GEAR_PARAMS)
  Constant4/1 -> MATLAB Function/8(BEAR_PARAMS)
  Constant5/1 -> MATLAB Function/9(IMB_PARAMS)
  Constant6/1 -> MATLAB Function/10(ENC_PARAMS)
  Constant7/1 -> MATLAB Function/11(t_noise)
  Constant8/1 -> MATLAB Function/12(enc_noise_signal)

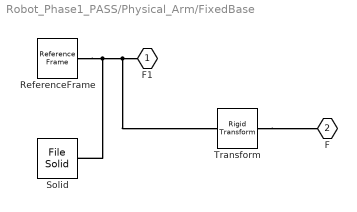
== system Robot_Phase1_PASS/Physical_Arm/FixedBase ==
  ReferenceFrame : sm_lib/Frames and Transforms/Reference Frame
  Solid : sm_lib/Body Elements/File Solid  ExtGeomFileName=base_Default_sldprt.STEP  UnitType=FromFile  ExtGeomFileUnits=m  StepReaderType=HEX  ExportConvexHullGeometry=off  InertiaType=Custom  BasedOnType=DensityFromFile  Density=1000  DensityUnits=kg/m^3  Mass=smiData.Solid(3).mass  MassUnits=kg  CenterOfMass=smiData.Solid(3).CoM  CenterOfMassUnits=mm  MomentsOfInertia=smiData.Solid(3).MoI  MomentsOfInertiaUnits=kg*mm^2  ProductsOfInertia=smiData.Solid(3).PoI  ProductsOfInertiaUnits=kg*mm^2  GraphicType=FromGeometry  MarkerShape=Sphere  MarkerSize=10  GraphicVisPropType=SimpleVisualProperties  GraphicDiffuseColor=smiData.Solid(3).color  GraphicOpacity=smiData.Solid(3).opacity  GraphicSpecularColor=[0.5 0.5 0.5 1.0]  GraphicAmbientColor=[0.15 0.15 0.15 1.0]  GraphicEmissiveColor=[0.0 0.0 0.0 1.0]  GraphicShininess=75  DoExposeReferenceFrame=on  SerializedFrames=<Frames/>
  Transform : sm_lib/Frames and Transforms/Rigid Transform  RotationMethod=ArbitraryAxis  FollAlignAxisA=+X  BaseAlignAxisA=+Y  FollAlignAxisB=+Y  BaseAlignAxisB=+Z  RotationStandardAxis=+X  RotationAngle=smiData.RigidTransform(6).angle  RotationAngleUnits=rad  RotationArbitraryAxis=smiData.RigidTransform(6).axis  RotationSequenceAxes=FollowerAxes  RotationSequence=XYX  RotationSequenceAngles=[0 0 0]  RotationSequenceAnglesUnits=deg  RotationMatrix=[1 0 0;0 1 0;0 0 1]  Quaternion=[1 0 0 0]  TranslationMethod=Cartesian  TranslationCartesianOffset=smiData.RigidTransform(6).translation  TranslationCartesianOffsetUnits=mm  TranslationStandardAxis=+Z  TranslationStandardOffset=0  TranslationStandardOffsetUnits=m  TranslationROffset=0  TranslationROffsetUnits=m  TranslationThetaOffset=0  TranslationThetaOffsetUnits=deg  TranslationZOffset=0  TranslationZOffsetUnits=m
  F1 : PMIOPort  Side=Left
  F : PMIOPort  Port=2  Side=Left
  connections:
  Solid/RConn1 -- ReferenceFrame/RConn1 -- Transform/LConn1 -- F1/RConn1
  Transform/RConn1 -- F/RConn1

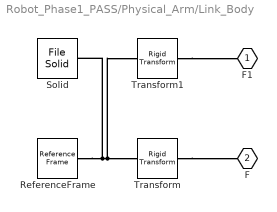
== system Robot_Phase1_PASS/Physical_Arm/Link_Body ==
  ReferenceFrame : sm_lib/Frames and Transforms/Reference Frame
  Solid : sm_lib/Body Elements/File Solid  ExtGeomFileName=Link1_Default_sldprt.STEP  UnitType=FromFile  ExtGeomFileUnits=m  StepReaderType=HEX  ExportConvexHullGeometry=off  InertiaType=Custom  BasedOnType=DensityFromFile  Density=1000  DensityUnits=kg/m^3  Mass=smiData.Solid(4).mass  MassUnits=kg  CenterOfMass=smiData.Solid(4).CoM  CenterOfMassUnits=mm  MomentsOfInertia=smiData.Solid(4).MoI  MomentsOfInertiaUnits=kg*mm^2  ProductsOfInertia=smiData.Solid(4).PoI  ProductsOfInertiaUnits=kg*mm^2  GraphicType=FromGeometry  MarkerShape=Sphere  MarkerSize=10  GraphicVisPropType=SimpleVisualProperties  GraphicDiffuseColor=smiData.Solid(4).color  GraphicOpacity=smiData.Solid(4).opacity  GraphicSpecularColor=[0.5 0.5 0.5 1.0]  GraphicAmbientColor=[0.15 0.15 0.15 1.0]  GraphicEmissiveColor=[0.0 0.0 0.0 1.0]  GraphicShininess=75  DoExposeReferenceFrame=on  SerializedFrames=<Frames/>
  Transform : sm_lib/Frames and Transforms/Rigid Transform  RotationMethod=ArbitraryAxis  FollAlignAxisA=+X  BaseAlignAxisA=+Y  FollAlignAxisB=+Y  BaseAlignAxisB=+Z  RotationStandardAxis=+Y  RotationAngle=smiData.RigidTransform(1).angle  RotationAngleUnits=rad  RotationArbitraryAxis=smiData.RigidTransform(1).axis  RotationSequenceAxes=FollowerAxes  RotationSequence=XYX  RotationSequenceAngles=[0 0 0]  RotationSequenceAnglesUnits=deg  RotationMatrix=[1 0 0;0 1 0;0 0 1]  Quaternion=[1 0 0 0]  TranslationMethod=Cartesian  TranslationCartesianOffset=smiData.RigidTransform(1).translation  TranslationCartesianOffsetUnits=mm  TranslationStandardAxis=+Z  TranslationStandardOffset=0  TranslationStandardOffsetUnits=m  TranslationROffset=0  TranslationROffsetUnits=m  TranslationThetaOffset=0  TranslationThetaOffsetUnits=deg  TranslationZOffset=0  TranslationZOffsetUnits=m
  Transform1 : sm_lib/Frames and Transforms/Rigid Transform  RotationMethod=ArbitraryAxis  FollAlignAxisA=+X  BaseAlignAxisA=+Y  FollAlignAxisB=+Y  BaseAlignAxisB=+Z  RotationStandardAxis=+X  RotationAngle=smiData.RigidTransform(4).angle  RotationAngleUnits=rad  RotationArbitraryAxis=smiData.RigidTransform(4).axis  RotationSequenceAxes=FollowerAxes  RotationSequence=XYX  RotationSequenceAngles=[0 0 0]  RotationSequenceAnglesUnits=deg  RotationMatrix=[1 0 0;0 1 0;0 0 1]  Quaternion=[1 0 0 0]  TranslationMethod=Cartesian  TranslationCartesianOffset=smiData.RigidTransform(4).translation  TranslationCartesianOffsetUnits=mm  TranslationStandardAxis=+Z  TranslationStandardOffset=0  TranslationStandardOffsetUnits=m  TranslationROffset=0  TranslationROffsetUnits=m  TranslationThetaOffset=0  TranslationThetaOffsetUnits=deg  TranslationZOffset=0  TranslationZOffsetUnits=m
  F1 : PMIOPort  Side=Left
  F : PMIOPort  Port=2  Side=Right
  connections:
  Solid/RConn1 -- ReferenceFrame/RConn1 -- Transform/LConn1 -- Transform1/LConn1
  Transform/RConn1 -- F/RConn1
  Transform1/RConn1 -- F1/RConn1

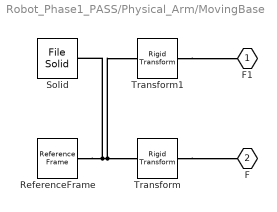
== system Robot_Phase1_PASS/Physical_Arm/MovingBase ==
  ReferenceFrame : sm_lib/Frames and Transforms/Reference Frame
  Solid : sm_lib/Body Elements/File Solid  ExtGeomFileName=base_joint_Default_sldprt.STEP  UnitType=FromFile  ExtGeomFileUnits=m  StepReaderType=HEX  ExportConvexHullGeometry=off  InertiaType=Custom  BasedOnType=DensityFromFile  Density=1000  DensityUnits=kg/m^3  Mass=smiData.Solid(1).mass  MassUnits=kg  CenterOfMass=smiData.Solid(1).CoM  CenterOfMassUnits=mm  MomentsOfInertia=smiData.Solid(1).MoI  MomentsOfInertiaUnits=kg*mm^2  ProductsOfInertia=smiData.Solid(1).PoI  ProductsOfInertiaUnits=kg*mm^2  GraphicType=FromGeometry  MarkerShape=Sphere  MarkerSize=10  GraphicVisPropType=SimpleVisualProperties  GraphicDiffuseColor=smiData.Solid(1).color  GraphicOpacity=smiData.Solid(1).opacity  GraphicSpecularColor=[0.5 0.5 0.5 1.0]  GraphicAmbientColor=[0.15 0.15 0.15 1.0]  GraphicEmissiveColor=[0.0 0.0 0.0 1.0]  GraphicShininess=75  DoExposeReferenceFrame=on  SerializedFrames=<Frames/>
  Transform : sm_lib/Frames and Transforms/Rigid Transform  RotationMethod=ArbitraryAxis  FollAlignAxisA=+X  BaseAlignAxisA=+Y  FollAlignAxisB=+Y  BaseAlignAxisB=+Z  RotationStandardAxis=-Y  RotationAngle=smiData.RigidTransform(3).angle  RotationAngleUnits=rad  RotationArbitraryAxis=smiData.RigidTransform(3).axis  RotationSequenceAxes=FollowerAxes  RotationSequence=XYX  RotationSequenceAngles=[0 0 0]  RotationSequenceAnglesUnits=deg  RotationMatrix=[1 0 0;0 1 0;0 0 1]  Quaternion=[1 0 0 0]  TranslationMethod=Cartesian  TranslationCartesianOffset=smiData.RigidTransform(3).translation  TranslationCartesianOffsetUnits=mm  TranslationStandardAxis=+Z  TranslationStandardOffset=0  TranslationStandardOffsetUnits=m  TranslationROffset=0  TranslationROffsetUnits=m  TranslationThetaOffset=0  TranslationThetaOffsetUnits=deg  TranslationZOffset=0  TranslationZOffsetUnits=m
  Transform1 : sm_lib/Frames and Transforms/Rigid Transform  RotationMethod=ArbitraryAxis  FollAlignAxisA=+X  BaseAlignAxisA=+Y  FollAlignAxisB=+Y  BaseAlignAxisB=+Z  RotationStandardAxis=+Y  RotationAngle=smiData.RigidTransform(5).angle  RotationAngleUnits=rad  RotationArbitraryAxis=smiData.RigidTransform(5).axis  RotationSequenceAxes=FollowerAxes  RotationSequence=XYX  RotationSequenceAngles=[0 0 0]  RotationSequenceAnglesUnits=deg  RotationMatrix=[1 0 0;0 1 0;0 0 1]  Quaternion=[1 0 0 0]  TranslationMethod=Cartesian  TranslationCartesianOffset=smiData.RigidTransform(5).translation  TranslationCartesianOffsetUnits=mm  TranslationStandardAxis=+Z  TranslationStandardOffset=0  TranslationStandardOffsetUnits=m  TranslationROffset=0  TranslationROffsetUnits=m  TranslationThetaOffset=0  TranslationThetaOffsetUnits=deg  TranslationZOffset=0  TranslationZOffsetUnits=m
  F1 : PMIOPort  Side=Right
  F : PMIOPort  Port=2  Side=Right
  connections:
  Solid/RConn1 -- ReferenceFrame/RConn1 -- Transform/LConn1 -- Transform1/LConn1
  Transform/RConn1 -- F/RConn1
  Transform1/RConn1 -- F1/RConn1

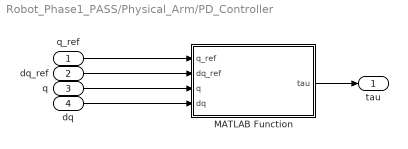
== system Robot_Phase1_PASS/Physical_Arm/PD_Controller ==
  q_ref : Inport
  dq_ref : Inport  Port=2
  q : Inport  Port=3
  dq : Inport  Port=4
  MATLAB Function : MATLAB Function  TreatAsAtomicUnit=on
  tau : Outport
  wires:
  MATLAB Function/1(tau) -> tau/1
  dq_ref/1 -> MATLAB Function/2(dq_ref)
  q_ref/1 -> MATLAB Function/1(q_ref)
  q/1 -> MATLAB Function/3(q)
  dq/1 -> MATLAB Function/4(dq)

== system Robot_Phase1_PASS/Virtual_Twin/End_Body ==
  ReferenceFrame : sm_lib/Frames and Transforms/Reference Frame
  Solid : sm_lib/Body Elements/File Solid  ExtGeomFileName=Link2_Default_sldprt.STEP  UnitType=FromFile  ExtGeomFileUnits=m  StepReaderType=HEX  ExportConvexHullGeometry=off  InertiaType=Custom  BasedOnType=DensityFromFile  Density=1000  DensityUnits=kg/m^3  Mass=sim_payload_mass  MassUnits=kg  CenterOfMass=[0, 0, 0]  CenterOfMassUnits=mm  MomentsOfInertia=[500, 500,500]  MomentsOfInertiaUnits=kg*mm^2  ProductsOfInertia=[0, 0, 0]  ProductsOfInertiaUnits=kg*mm^2  GraphicType=FromGeometry  MarkerShape=Sphere  MarkerSize=10  GraphicVisPropType=SimpleVisualProperties  GraphicDiffuseColor=smiData.Solid(2).color  GraphicOpacity=smiData.Solid(2).opacity  GraphicSpecularColor=[0.5 0.5 0.5 1.0]  GraphicAmbientColor=[0.15 0.15 0.15 1.0]  GraphicEmissiveColor=[0.0 0.0 0.0 1.0]  GraphicShininess=75  DoExposeReferenceFrame=on  SerializedFrames=<Frames/>
  Transform : sm_lib/Frames and Transforms/Rigid Transform  RotationMethod=ArbitraryAxis  FollAlignAxisA=+X  BaseAlignAxisA=+Y  FollAlignAxisB=+Y  BaseAlignAxisB=+Z  RotationStandardAxis=+X  RotationAngle=smiData.RigidTransform(2).angle  RotationAngleUnits=rad  RotationArbitraryAxis=smiData.RigidTransform(2).axis  RotationSequenceAxes=FollowerAxes  RotationSequence=XYX  RotationSequenceAngles=[0 0 0]  RotationSequenceAnglesUnits=deg  RotationMatrix=[1 0 0;0 1 0;0 0 1]  Quaternion=[1 0 0 0]  TranslationMethod=Cartesian  TranslationCartesianOffset=smiData.RigidTransform(2).translation  TranslationCartesianOffsetUnits=mm  TranslationStandardAxis=+Z  TranslationStandardOffset=0  TranslationStandardOffsetUnits=m  TranslationROffset=0  TranslationROffsetUnits=m  TranslationThetaOffset=0  TranslationThetaOffsetUnits=deg  TranslationZOffset=0  TranslationZOffsetUnits=m
  F : PMIOPort  Side=Left
  connections:
  Solid/RConn1 -- ReferenceFrame/RConn1 -- Transform/LConn1
  Transform/RConn1 -- F/RConn1
